simulink model "smg"  (Simulink 2.00)
settings: Solver=ode45  StartTime=0.0  StopTime=tstop  MaxStep=1e-2  RelTol=1e-5  AbsTol=1e-6
values from neighbouring files (symbols this model uses):
  I = [ 0 0.0112 0.0310 0.0585 0.0740 0.0895 0.1084 0.1153 0.1308 0.1437 0.1583 0.1686 0.1841 0.2004 0.2142 0.2331 0.2477 0.2753 0.2933 0.3131 0.3381 0.3639 0.3828 0.4000]    [MGINIT.M]
  ifull = [-1.*iud' i]    [MGINIT.M]
  Ifull = sqrt(2).*[-1.*Iud' I]    [MGINIT.M]
  psifull = [-1.*psiud' psi]    [MGINIT.M]
  tstop = 0.2    [M1.M]    (also in M4.M = 1.2; MGINIT.M = 3.5)
  V = [ 0.00 7.40 20.50 37.30 47.31 57.12 68.85 72.80 81.19 87.82 95.46 100.7 107.04 112.37 116.04 119.75 121.92 125.61 127.92 130.25 132.53 134.85 136.1 137.5 ]    [MGINIT.M]
  Vfull = sqrt(2).*[-1.*Vud' V]    [MGINIT.M]
  Vmaxrms = V(nV-1)    [MGINIT.M]
  we = 377    [MGINIT.M]
settings Model: SaveTime=off  SaveOutput=off  ConsistencyChecking=off

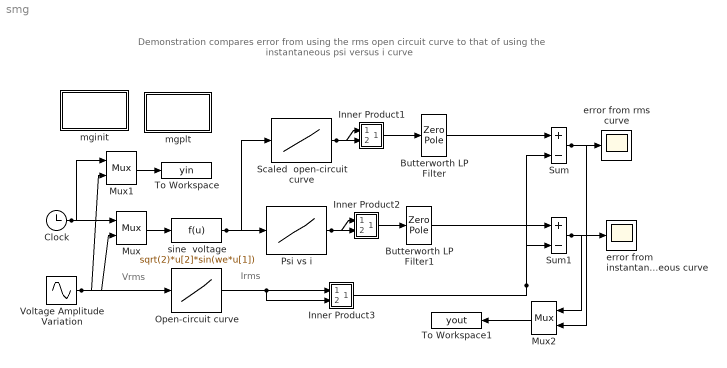
== system smg ==
  note: Vrms
  note: Demonstration compares error from using the rms open circuit curve
      | to that of using the instantaneous psi versus i curve
  note: Irms
  Butterworth LP Filter : ZeroPole  Zeros=z  Poles=p  Gain=k  mask(buttap){@1=300, @2=4}
      mask prompts: @1 "Cutoff frequency (rad/sec)"; @2 "Order"
      mask help:
      | Analog Butterworth low pass filter.
      |
      | (Requires Signal Processing Toolbox)
      mask init:
      | [z,p,k]=buttap(@2); z=@1*z; p=@1*p; k=real(prod(-p)); [num,den]=zp2tf(z,p,k); w=logspace(log10(@1/10),log10(10*@1),20); h=freqs(num,den,w);
      mask Help: Butterworth low pass filter using MATLAB's butter command.
      mask Display: plot(20*log10(w),20*log10(abs(h)))
  Butterworth LP Filter1 : ZeroPole  Zeros=z  Poles=p  Gain=k  mask(buttap){@1=300, @2=4}
      mask prompts: @1 "Cutoff frequency (rad/sec)"; @2 "Order"
      mask help:
      | Analog Butterworth low pass filter.
      |
      | (Requires Signal Processing Toolbox)
      mask init:
      | [z,p,k]=buttap(@2); z=@1*z; p=@1*p; k=real(prod(-p)); [num,den]=zp2tf(z,p,k); w=logspace(log10(@1/10),log10(10*@1),20); h=freqs(num,den,w);
      mask Help: Butterworth low pass filter using MATLAB's butter command.
      mask Display: plot(20*log10(w),20*log10(abs(h)))
  Clock : Clock
      settings: DeleteFcn=simclock BlockIsBeingDestroyed  PostSaveFcn=simclock Save
  Inner Product1 : Subsystem
      mask Type: Dot Product
      mask Description:
      | Inner (dot) product.
      | y=sum(u1.*u2)
      mask Help: Computes the inner (dot) product of the inputs: sum(u1.*u2).  The inputs are vectors of the same length. Output is a scalar.
      mask Display: disp('.\n')
  Inner Product2 : Subsystem
      mask Type: Dot Product
      mask Description:
      | Inner (dot) product.
      | y=sum(u1.*u2)
      mask Help: Computes the inner (dot) product of the inputs: sum(u1.*u2).  The inputs are vectors of the same length. Output is a scalar.
      mask Display: disp('.\n')
  Inner Product3 : Subsystem
      mask Type: Dot Product
      mask Description:
      | Inner (dot) product.
      | y=sum(u1.*u2)
      mask Help: Computes the inner (dot) product of the inputs: sum(u1.*u2).  The inputs are vectors of the same length. Output is a scalar.
      mask Display: disp('.\n')
  mginit : Subsystem
      settings: OpenFcn=mginit
      mask Type: Masked block of mginit.m
      mask Help: Uses mginit.m to initialize simulation
      mask Display: disp('Initialize')
  mgplt : Subsystem
      settings: OpenFcn=mgplt
      mask Type: Masked block of mgplt.m
      mask Help: Uses mgplt.m to plot results
      mask Display: disp('Plot')
  Mux : Mux  Inputs=2
  Mux1 : Mux  Inputs=2
  Mux2 : Mux  Orientation=left  Inputs=2
  Open-circuit curve : Lookup  InputValues=V  OutputValues=I
  Psi vs i : Lookup  InputValues=psifull  OutputValues=ifull
  Scaled  open-circuit curve : Lookup  InputValues=Vfull  OutputValues=Ifull
  Sum : Sum  Inputs=+-
  Sum1 : Sum  Inputs=+-
  To Workspace : ToWorkspace  VariableName=yin  SampleTime=0
      settings: Buffer=4000
  To Workspace1 : ToWorkspace  VariableName=yout  SampleTime=0
      settings: Buffer=4000
  Voltage Amplitude Variation : Sin  Amplitude=Vmaxrms  Frequency=pi/tstop  Phase=0  SampleTime=-1
  error from rms curve : Scope
      settings: TickLabels=on  TimeRange=3.500000  YMin=-0.100000  YMax=0.100000  SaveToWorkspace=off  SaveName=ScopeData
  error from  instantaneous curve : Scope
      settings: TickLabels=on  TimeRange=3.500000  YMin=-0.100000  YMax=0.100000  SaveToWorkspace=off  SaveName=ScopeData
  sine  voltage : Fcn  Expr=sqrt(2)*u[2]*sin(we*u[1])
  wires:
  Inner Product3/1(out_1) -> Sum/2, Sum1/2
  Open-circuit curve/1 -> Inner Product3/2(in_2), Inner Product3/1(in_1)
  Butterworth LP Filter/1 -> Sum/1
  Butterworth LP Filter1/1 -> Sum1/1
  Mux/1 -> sine  voltage/1
  Voltage Amplitude Variation/1 -> Mux/2, Open-circuit curve/1, Mux1/2
  sine  voltage/1 -> Psi vs i/1, Scaled  open-circuit curve/1
  Inner Product2/1(out_1) -> Butterworth LP Filter1/1
  Inner Product1/1(out_1) -> Butterworth LP Filter/1
  Scaled  open-circuit curve/1 -> Inner Product1/1(in_1), Inner Product1/2(in_2)
  Psi vs i/1 -> Inner Product2/1(in_1), Inner Product2/2(in_2)
  Mux1/1 -> To Workspace/1
  Clock/1 -> Mux/1, Mux1/1
  Sum1/1 -> error from  instantaneous curve/1, Mux2/1
  Sum/1 -> error from rms curve/1, Mux2/2
  Mux2/1 -> To Workspace1/1

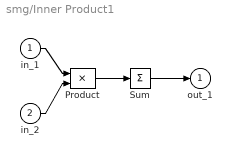
== system smg/Inner Product1 ==
  in_1 : Inport  Port=1  PortWidth=-1  SampleTime=-1
  in_2 : Inport  Port=2  PortWidth=-1  SampleTime=-1
  Product : Product  Inputs=2
  Sum : Sum  Inputs=+
  out_1 : Outport  Port=1  InitialOutput=0
  wires:
  in_2/1 -> Product/2
  in_1/1 -> Product/1
  Product/1 -> Sum/1
  Sum/1 -> out_1/1

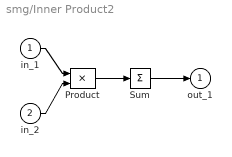
== system smg/Inner Product2 ==
  in_1 : Inport  Port=1  PortWidth=-1  SampleTime=-1
  in_2 : Inport  Port=2  PortWidth=-1  SampleTime=-1
  Product : Product  Inputs=2
  Sum : Sum  Inputs=+
  out_1 : Outport  Port=1  InitialOutput=0
  wires:
  in_2/1 -> Product/2
  in_1/1 -> Product/1
  Product/1 -> Sum/1
  Sum/1 -> out_1/1

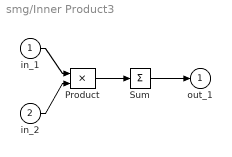
== system smg/Inner Product3 ==
  in_1 : Inport  Port=1  PortWidth=-1  SampleTime=-1
  in_2 : Inport  Port=2  PortWidth=-1  SampleTime=-1
  Product : Product  Inputs=2
  Sum : Sum  Inputs=+
  out_1 : Outport  Port=1  InitialOutput=0
  wires:
  in_2/1 -> Product/2
  in_1/1 -> Product/1
  Product/1 -> Sum/1
  Sum/1 -> out_1/1

== system smg/mginit ==
  note: Masked block of mginit.m

== system smg/mgplt ==
  note: Masked block of mgplt.m
